simulink model "schema3"  (R2020b)
settings: Solver=VariableStepAuto  StartTime=0.0  StopTime=10.0  RelTol=1e-3
values from neighbouring files (symbols this model uses):
  DenC = [1]    [TP2.m]    (also in ptschema2.m; ptschema3.m)
  DenG = [1/(16.89*50) 1/16.89 0]    [TP2.m]    (also in ptschema2.m = [1/(16.89*50)  1/16.89 0]; ptschema3.m)
  Fve = 1    [TP2.m]    (also in ptschema2.m; ptschema3.m)
  FvPs = 1    [TP2.m]    (also in ptschema2.m; ptschema3.m)
  FvPu = 1    [TP2.m]    (also in ptschema2.m; ptschema3.m)
  Ive = 0    [TP2.m]    (also in ptschema2.m; ptschema3.m)
  IvPs = 0    [TP2.m]    (also in ptschema2.m; ptschema3.m)
  IvPu = 0    [TP2.m]    (also in ptschema2.m; ptschema3.m)
  NumC = [1]    [TP2.m]    (also in ptschema2.m; ptschema3.m)
  NumG = [1]    [TP2.m]    (also in ptschema2.m; ptschema3.m)
  SampleTime = 0.001    [ptschema3.m]
  Stepte = 0    [TP2.m]    (also in ptschema2.m; ptschema3.m)
  SteptPs = 10    [TP2.m]    (also in ptschema2.m; ptschema3.m)
  SteptPu = 5    [TP2.m]    (also in ptschema2.m; ptschema3.m)
settings Model: Creator=Antoine  LastModifiedBy=Antoine

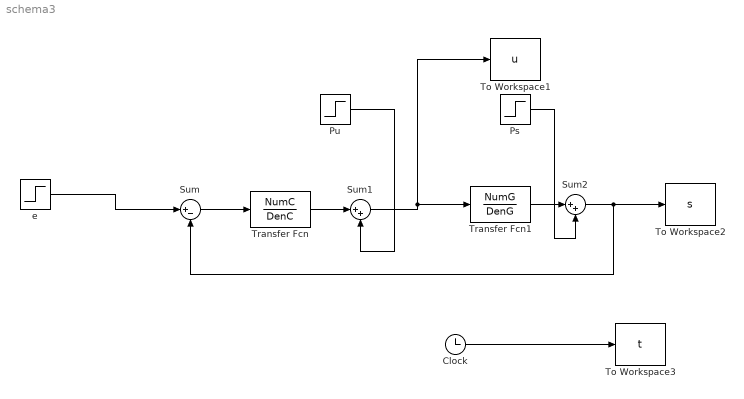
== system schema3 ==
  Clock : Clock
  Ps : Step  Time=SteptPs  Before=IvPs  After=FvPs  SampleTime=0
  Pu : Step  Time=SteptPu  Before=IvPu  After=FvPu  SampleTime=0
  Sum : Sum  Inputs=|+-
  Sum1 : Sum  Inputs=|++
  Sum2 : Sum  Inputs=|++
  To Workspace1 : ToWorkspace  VariableName=u  SampleTime=SampleTime
      settings: MaxDataPoints=DataHistory  Save2DSignal=2-D array (concatenate along first dimension)
  To Workspace2 : ToWorkspace  VariableName=s  SampleTime=SampleTime
      settings: MaxDataPoints=DataHistory  Save2DSignal=2-D array (concatenate along first dimension)
  To Workspace3 : ToWorkspace  VariableName=t  SampleTime=SampleTime
      settings: MaxDataPoints=DataHistory  Save2DSignal=2-D array (concatenate along first dimension)
  Transfer Fcn : TransferFcn  Numerator=NumC  Denominator=DenC
  Transfer Fcn1 : TransferFcn  Numerator=NumG  Denominator=DenG
  e : Step  Time=Stepte  Before=Ive  After=Fve  SampleTime=0
  wires:
  Sum/1 -> Transfer Fcn/1
  Transfer Fcn/1 -> Sum1/1
  Pu/1 -> Sum1/2
  Sum1/1 -> To Workspace1/1, Transfer Fcn1/1
  Transfer Fcn1/1 -> Sum2/1
  Sum2/1 -> To Workspace2/1, Sum/2
  Ps/1 -> Sum2/2
  e/1 -> Sum/1
  Clock/1 -> To Workspace3/1
